simulink model "C172S_HeadingHold_V1"  (R2026a)
settings: Solver=ode4  StartTime=0  StopTime=100  FixedStep=0.01
InitFcn:
  | hh1Data = c172sLateralDirectionalData();
  | [~,hh1Plant] = c172sLateralDirectionalPlant(hh1Data);
  | hh1YawController = c172sYawDamperData();
  | hh1RudderActuator = c172sRudderActuatorData();
  | hh1RollController = c172sRollAttitudeControllerData();
  | hh1AileronActuator = c172sAileronActuatorData();
  | hh1HeadingSensor = c172sHeadingSensorData();
  | hh1HeadingController = c172sHeadingHoldControllerData();
  | if ~strcmp(hh1Data.model.version,hh1HeadingController.requiredPlantVersion), error('HH V1 plant dependency mismatch.'); end
  | if ~strcmp(hh1YawController.artifactRevision,hh1HeadingController.requiredYawDamperRevision), error('HH V1 yaw-controller dependency mismatch.'); end
  | if ~strcmp(hh1RudderActuator.artifactRevision,hh1HeadingController.requiredRudderAuditRevision), error('HH V1 rudder-audit dependency mismatch.'); end
  | if ~strcmp(hh1AileronActuator.artifactRevision,hh1HeadingController.requiredAileronAuditRevision), error('HH V1 aileron-audit dependency mismatch.'); end
  | if ~strcmp(hh1RollController.artifactRevision,hh1HeadingController.requiredRollControllerRevision), error('HH V1 roll-controller dependency mismatch.'); end
  | if ~strcmp(hh1HeadingSensor.artifactRevision,hh1HeadingController.requiredHeadingSensorRevision), error('HH V1 heading-sensor dependency mismatch.'); end
  | A_hh1 = hh1Plant.A; B_hh1 = hh1Plant.B;
  | C_hh1 = hh1Plant.C; D_hh1 = hh1Plant.D;
  | Kphi_hh1 = hh1RollController.bankProportionalGain;
  | Ki_hh1 = hh1RollController.bankIntegralGain_per_s;
  | Kp_hh1 = hh1RollController.rollRateGain_s;
  | Tcmd_hh1 = hh1RollController.commandFilterTimeConstant_s;
  | Kr_hh1 = hh1YawController.rudderGain_s;
  | Tw_hh1 = hh1YawController.washoutTimeConstant_s;
  | TsRudder_hh1 = hh1RudderActuator.sensor.filterTimeConstant_s;
  | tauRudder_hh1 = hh1RudderActuator.dynamics.timeConstant_s;
  | TsRoll_hh1 = hh1AileronActuator.sensor.filterTimeConstant_s;
  | tauAileron_hh1 = hh1AileronActuator.dynamics.timeConstant_s;
  | Tt_hh1 = hh1AileronActuator.antiWindup.trackingTimeConstant_s;
  | delaySampleTime_hh1 = hh1AileronActuator.sensor.nominalDelay_s;
  | Kpsi_hh1 = hh1HeadingController.headingErrorGain;
  | TsHeading_hh1 = hh1HeadingSensor.filterTimeConstant_s;
  | headingDelaySampleTime_hh1 = hh1HeadingSensor.nominalDelay_s/5;
  | bankCommandLower_hh1_rad = -deg2rad(hh1HeadingController.bankCommandAuthority_deg);
  | bankCommandUpper_hh1_rad = deg2rad(hh1HeadingController.bankCommandAuthority_deg);
  | autoAileronLower_hh1_rad = hh1AileronActuator.authority.lowerLimit_rad;
  | autoAileronUpper_hh1_rad = hh1AileronActuator.authority.upperLimit_rad;
  | aileronRateLower_hh1_radps = -deg2rad(hh1AileronActuator.dynamics.rateLimit_degps);
  | aileronRateUpper_hh1_radps = deg2rad(hh1AileronActuator.dynamics.rateLimit_degps);
  | totalAileronLower_hh1_rad = hh1AileronActuator.physicalTravel.lowerLimit_rad;
  | totalAileronUpper_hh1_rad = hh1AileronActuator.physicalTravel.upperLimit_rad;
  | autoRudderLower_hh1_rad = hh1RudderActuator.authority.lowerLimit_rad;
  | autoRudderUpper_hh1_rad = hh1RudderActuator.authority.upperLimit_rad;
  | rudderRateLower_hh1_radps = -deg2rad(hh1RudderActuator.dynamics.rateLimit_degps);
  | rudderRateUpper_hh1_radps = deg2rad(hh1RudderActuator.dynamics.rateLimit_degps);
  | totalRudderLower_hh1_rad = hh1RudderActuator.physicalTravel.lowerLimit_rad;
  | totalRudderUpper_hh1_rad = hh1RudderActuator.physicalTravel.upperLimit_rad;
  | if ~exist('headingCommand_hh1_rad','var'), headingCommand_hh1_rad = deg2rad(30); end
  | if ~exist('headingBias_hh1_rad','var'), headingBias_hh1_rad = 0; end
  | if ~exist('headingNoiseAmplitude_hh1_rad','var'), headingNoiseAmplitude_hh1_rad = 0; end
  | if ~exist('headingNoiseFrequency_hh1_radps','var'), headingNoiseFrequency_hh1_radps = 0.8; end
  | if ~exist('pilotAileronBias_hh1_rad','var'), pilotAileronBias_hh1_rad = 0; end
  | if ~exist('pilotAileronPulse_hh1_rad','var'), pilotAileronPulse_hh1_rad = 0; end
  | if ~exist('pilotRudderBias_hh1_rad','var'), pilotRudderBias_hh1_rad = 0; end
  | if ~exist('pilotRudderPulse_hh1_rad','var'), pilotRudderPulse_hh1_rad = 0; end
  | if ~exist('aileronPulseStart_hh1_s','var'), aileronPulseStart_hh1_s = 5; end
  | if ~exist('aileronPulseEnd_hh1_s','var'), aileronPulseEnd_hh1_s = 6; end
  | if ~exist('rudderPulseStart_hh1_s','var'), rudderPulseStart_hh1_s = 5; end
  | if ~exist('rudderPulseEnd_hh1_s','var'), rudderPulseEnd_hh1_s = 6; end
  | if ~exist('pNoiseAmplitude_hh1_radps','var'), pNoiseAmplitude_hh1_radps = 0; end
  | if ~exist('pNoiseFrequency_hh1_radps','var'), pNoiseFrequency_hh1_radps = 50; end
  | if ~exist('phiNoiseAmplitude_hh1_rad','var'), phiNoiseAmplitude_hh1_rad = 0; end
  | if ~exist('phiNoiseFrequency_hh1_radps','var'), phiNoiseFrequency_hh1_radps = 5; end
  | if ~exist('yawNoiseAmplitude_hh1_radps','var'), yawNoiseAmplitude_hh1_radps = 0; end
  | if ~exist('yawNoiseFrequency_hh1_radps','var'), yawNoiseFrequency_hh1_radps = 50; end
  | if ~exist('antiWindupEnable_hh1','var'), antiWindupEnable_hh1 = 1; end
  | if ~exist('x0_hh1','var'), x0_hh1 = zeros(5,1); end
  | if ~exist('rDelay0_hh1_radps','var'), rDelay0_hh1_radps = x0_hh1(3); end
  | if ~exist('pDelay0_hh1_radps','var'), pDelay0_hh1_radps = x0_hh1(2); end
  | if ~exist('phiDelay0_hh1_rad','var'), phiDelay0_hh1_rad = x0_hh1(4); end
  | if ~exist('rSensor0_hh1_radps','var'), rSensor0_hh1_radps = 0; end
  | if ~exist('xw0_hh1_radps','var'), xw0_hh1_radps = 0; end
  | if ~exist('deltaRAuto0_hh1_rad','var'), deltaRAuto0_hh1_rad = 0; end
  | if ~exist('pSensor0_hh1_radps','var'), pSensor0_hh1_radps = 0; end
  | if ~exist('phiSensor0_hh1_rad','var'), phiSensor0_hh1_rad = 0; end
  | if ~exist('psiDelay0_hh1_rad','var'), psiDelay0_hh1_rad = x0_hh1(5); end
  | if ~exist('psiSensor0_hh1_rad','var'), psiSensor0_hh1_rad = x0_hh1(5)+headingBias_hh1_rad; end
  | if ~exist('xi0_hh1_rad_s','var'), xi0_hh1_rad_s = 0; end
  | if ~exist('deltaAAuto0_hh1_rad','var'), deltaAAuto0_hh1_rad = 0; end
  | if ~exist('filteredCommand0_hh1_rad','var'), filteredCommand0_hh1_rad = 0; end
undefined symbols (not defined in the file or in its folder): aileronPulseEnd_hh1_s, aileronPulseStart_hh1_s, antiWindupEnable_hh1, deltaAAuto0_hh1_rad, deltaRAuto0_hh1_rad, filteredCommand0_hh1_rad, headingBias_hh1_rad, headingNoiseAmplitude_hh1_rad, headingNoiseFrequency_hh1_radps, pDelay0_hh1_radps, phiDelay0_hh1_rad, phiNoiseAmplitude_hh1_rad, phiNoiseFrequency_hh1_radps, phiSensor0_hh1_rad, pilotAileronBias_hh1_rad, pilotAileronPulse_hh1_rad, pilotRudderBias_hh1_rad, pilotRudderPulse_hh1_rad, pNoiseAmplitude_hh1_radps, pNoiseFrequency_hh1_radps, pSensor0_hh1_radps, psiDelay0_hh1_rad, psiSensor0_hh1_rad, rDelay0_hh1_radps, rSensor0_hh1_radps, rudderPulseEnd_hh1_s, rudderPulseStart_hh1_s, x0_hh1, xi0_hh1_rad_s, xw0_hh1_radps, yawNoiseAmplitude_hh1_radps, yawNoiseFrequency_hh1_radps
settings Model: Creator=Shahi  LastModifiedBy=Shahi

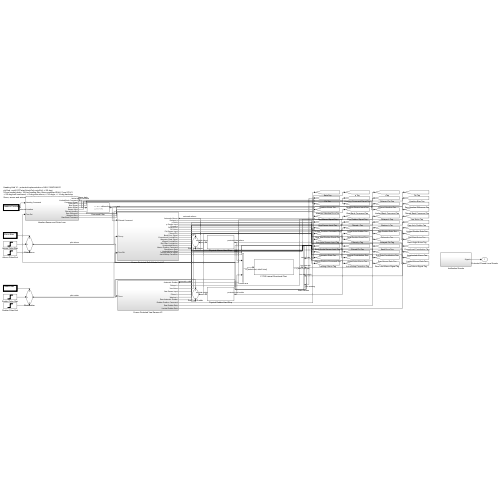
[thumbnail: Simulink's stored preview of the top-level diagram]
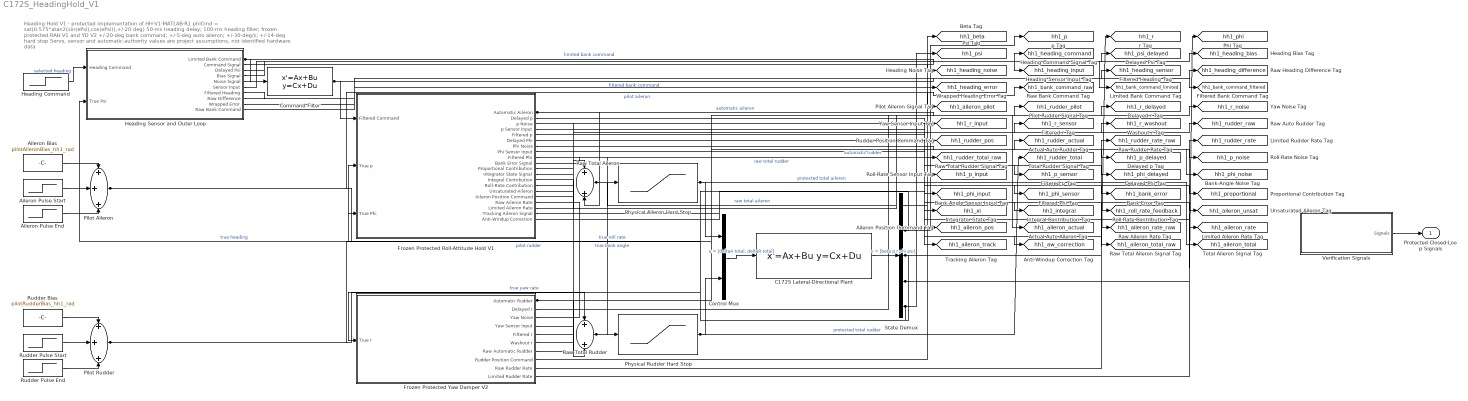
== system C172S_HeadingHold_V1 ==
  note: Heading Hold V1 - protected implementation of HH-V1-MATLAB-R1
      | phiCmd = sat(0.575*atan2(sin(ePsi),cos(ePsi)),+/-20 deg)
      | 50-ms heading delay; 100-ms heading filter; frozen protected RAH V1 and YD V2
      | +/-20-deg bank command; +/-5-deg auto aileron; +/-30-deg/s; +/-14-deg hard stop
      | Servo, sensor and automatic-authority values are project assumptions, not identified hardware data
  Aileron Bias : Constant  Value=pilotAileronBias_hh1_rad
  Aileron Pulse End : Step  Time=aileronPulseEnd_hh1_s  FinalValue=-pilotAileronPulse_hh1_rad  SampleTime=0
  Aileron Pulse Start : Step  Time=aileronPulseStart_hh1_s  FinalValue=pilotAileronPulse_hh1_rad  SampleTime=0
  C172S Lateral-Directional Plant : StateSpace  A=A_hh1  B=B_hh1  C=C_hh1  D=D_hh1  InitialCondition=x0_hh1
  Command Filter : StateSpace  A=-1/Tcmd_hh1  B=1/Tcmd_hh1  D=0  InitialCondition=filteredCommand0_hh1_rad
  Control Mux : Mux  Inputs=2
  Frozen Protected Roll-Attitude Hold V1 : Subsystem
  Frozen Protected Yaw Damper V2 : Subsystem
  Heading Command : Step  Time=0  FinalValue=headingCommand_hh1_rad  SampleTime=0
  Heading Sensor and Outer Loop : Subsystem
  Physical Aileron Hard Stop : Saturate  UpperLimit=totalAileronUpper_hh1_rad  LowerLimit=totalAileronLower_hh1_rad
  Physical Rudder Hard Stop : Saturate  UpperLimit=totalRudderUpper_hh1_rad  LowerLimit=totalRudderLower_hh1_rad
  Pilot Aileron : Sum  Inputs=+++
  Pilot Rudder : Sum  Inputs=+++
  Raw Total Aileron : Sum
  Raw Total Rudder : Sum
  Rudder Bias : Constant  Value=pilotRudderBias_hh1_rad
  Rudder Pulse End : Step  Time=rudderPulseEnd_hh1_s  FinalValue=-pilotRudderPulse_hh1_rad  SampleTime=0
  Rudder Pulse Start : Step  Time=rudderPulseStart_hh1_s  FinalValue=pilotRudderPulse_hh1_rad  SampleTime=0
  State Demux : Demux  Outputs=5
  Verification Signals : Subsystem
  Protected Closed-Loop Signals : Outport
  tag scope: hh1_aileron_actual=global, hh1_aileron_pilot=global, hh1_aileron_pos=global, hh1_aileron_rate=global, hh1_aileron_rate_raw=global, hh1_aileron_total=global, hh1_aileron_total_raw=global, hh1_aileron_track=global, hh1_aileron_unsat=global, hh1_aw_correction=global, hh1_bank_command_filtered=global, hh1_bank_command_limited=global, hh1_bank_command_raw=global, hh1_bank_error=global, hh1_beta=global, hh1_heading_bias=global, hh1_heading_command=global, hh1_heading_difference=global, hh1_heading_error=global, hh1_heading_input=global, hh1_heading_noise=global, hh1_heading_sensor=global, hh1_integral=global, hh1_p=global, hh1_p_delayed=global, hh1_p_input=global, hh1_p_noise=global, hh1_p_sensor=global, hh1_phi=global, hh1_phi_delayed=global, hh1_phi_input=global, hh1_phi_noise=global, hh1_phi_sensor=global, hh1_proportional=global, hh1_psi=global, hh1_psi_delayed=global, hh1_r=global, hh1_r_delayed=global, hh1_r_input=global, hh1_r_noise=global, hh1_r_sensor=global, hh1_r_washout=global, hh1_roll_rate_feedback=global, hh1_rudder_actual=global, hh1_rudder_pilot=global, hh1_rudder_pos=global, hh1_rudder_rate=global, hh1_rudder_rate_raw=global, hh1_rudder_raw=global, hh1_rudder_total=global, hh1_rudder_total_raw=global, hh1_xi=global
  wires:
  Heading Command/1 -> Heading Sensor and Outer Loop/1(Heading Command)  "selected heading"
  Heading Sensor and Outer Loop/1(Limited Bank Command) -> Command Filter/1, [hh1_bank_command_limited]  "limited bank command"
  Command Filter/1 -> Frozen Protected Roll-Attitude Hold V1/1(Filtered Command), [hh1_bank_command_filtered]  "filtered bank command"
  Aileron Bias/1 -> Pilot Aileron/1
  Aileron Pulse Start/1 -> Pilot Aileron/2
  Aileron Pulse End/1 -> Pilot Aileron/3
  Rudder Bias/1 -> Pilot Rudder/1
  Rudder Pulse Start/1 -> Pilot Rudder/2
  Rudder Pulse End/1 -> Pilot Rudder/3
  Pilot Aileron/1 -> Raw Total Aileron/1, [hh1_aileron_pilot]  "pilot aileron"
  Frozen Protected Roll-Attitude Hold V1/1(Automatic Aileron) -> Raw Total Aileron/2, [hh1_aileron_actual]  "automatic aileron"
  Raw Total Aileron/1 -> Physical Aileron Hard Stop/1, [hh1_aileron_total_raw]  "raw total aileron"
  Physical Aileron Hard Stop/1 -> Control Mux/1, [hh1_aileron_total]  "protected total aileron"
  Pilot Rudder/1 -> Raw Total Rudder/1, [hh1_rudder_pilot]  "pilot rudder"
  Frozen Protected Yaw Damper V2/1(Automatic Rudder) -> Raw Total Rudder/2, [hh1_rudder_actual]  "automatic rudder"
  Raw Total Rudder/1 -> Physical Rudder Hard Stop/1, [hh1_rudder_total_raw]  "raw total rudder"
  Physical Rudder Hard Stop/1 -> Control Mux/2, [hh1_rudder_total]  "protected total rudder"
  Control Mux/1 -> C172S Lateral-Directional Plant/1  "u = [deltaA total, deltaR total]"
  C172S Lateral-Directional Plant/1 -> State Demux/1  "x = [beta p r phi psi]"
  State Demux/2 -> Frozen Protected Roll-Attitude Hold V1/2(True p), [hh1_p]  "true roll rate"
  State Demux/4 -> Frozen Protected Roll-Attitude Hold V1/3(True Phi), [hh1_phi]  "true bank angle"
  State Demux/3 -> Frozen Protected Yaw Damper V2/1(True r), [hh1_r]  "true yaw rate"
  State Demux/5 -> Heading Sensor and Outer Loop/2(True Psi), [hh1_psi]  "true heading"
  Verification Signals/1(Signals) -> Protected Closed-Loop Signals/1
  State Demux/1 -> [hh1_beta]
  Heading Sensor and Outer Loop/2(Command Signal) -> [hh1_heading_command]
  Heading Sensor and Outer Loop/3(Delayed Psi) -> [hh1_psi_delayed]
  Heading Sensor and Outer Loop/4(Bias Signal) -> [hh1_heading_bias]
  Heading Sensor and Outer Loop/5(Noise Signal) -> [hh1_heading_noise]
  Heading Sensor and Outer Loop/6(Sensor Input) -> [hh1_heading_input]
  Heading Sensor and Outer Loop/7(Filtered Heading) -> [hh1_heading_sensor]
  Heading Sensor and Outer Loop/8(Raw Difference) -> [hh1_heading_difference]
  Heading Sensor and Outer Loop/9(Wrapped Error) -> [hh1_heading_error]
  Heading Sensor and Outer Loop/10(Raw Bank Command) -> [hh1_bank_command_raw]
  Frozen Protected Yaw Damper V2/2(Delayed r) -> [hh1_r_delayed]
  Frozen Protected Yaw Damper V2/3(Yaw Noise) -> [hh1_r_noise]
  Frozen Protected Yaw Damper V2/4(Yaw Sensor Input) -> [hh1_r_input]
  Frozen Protected Yaw Damper V2/5(Filtered r) -> [hh1_r_sensor]
  Frozen Protected Yaw Damper V2/6(Washout r) -> [hh1_r_washout]
  Frozen Protected Yaw Damper V2/7(Raw Automatic Rudder) -> [hh1_rudder_raw]
  Frozen Protected Yaw Damper V2/8(Rudder Position Command) -> [hh1_rudder_pos]
  Frozen Protected Yaw Damper V2/9(Raw Rudder Rate) -> [hh1_rudder_rate_raw]
  Frozen Protected Yaw Damper V2/10(Limited Rudder Rate) -> [hh1_rudder_rate]
  Frozen Protected Roll-Attitude Hold V1/2(Delayed p) -> [hh1_p_delayed]
  Frozen Protected Roll-Attitude Hold V1/3(p Noise) -> [hh1_p_noise]
  Frozen Protected Roll-Attitude Hold V1/4(p Sensor Input) -> [hh1_p_input]
  Frozen Protected Roll-Attitude Hold V1/5(Filtered p) -> [hh1_p_sensor]
  Frozen Protected Roll-Attitude Hold V1/6(Delayed Phi) -> [hh1_phi_delayed]
  Frozen Protected Roll-Attitude Hold V1/7(Phi Noise) -> [hh1_phi_noise]
  Frozen Protected Roll-Attitude Hold V1/8(Phi Sensor Input) -> [hh1_phi_input]
  Frozen Protected Roll-Attitude Hold V1/9(Filtered Phi) -> [hh1_phi_sensor]
  Frozen Protected Roll-Attitude Hold V1/10(Bank Error Signal) -> [hh1_bank_error]
  Frozen Protected Roll-Attitude Hold V1/11(Proportional Contribution) -> [hh1_proportional]
  Frozen Protected Roll-Attitude Hold V1/12(Integrator State Signal) -> [hh1_xi]
  Frozen Protected Roll-Attitude Hold V1/13(Integral Contribution) -> [hh1_integral]
  Frozen Protected Roll-Attitude Hold V1/14(Roll-Rate Contribution) -> [hh1_roll_rate_feedback]
  Frozen Protected Roll-Attitude Hold V1/15(Unsaturated Aileron) -> [hh1_aileron_unsat]
  Frozen Protected Roll-Attitude Hold V1/16(Aileron Position Command) -> [hh1_aileron_pos]
  Frozen Protected Roll-Attitude Hold V1/17(Raw Aileron Rate) -> [hh1_aileron_rate_raw]
  Frozen Protected Roll-Attitude Hold V1/18(Limited Aileron Rate) -> [hh1_aileron_rate]
  Frozen Protected Roll-Attitude Hold V1/19(Tracking Aileron Signal) -> [hh1_aileron_track]
  Frozen Protected Roll-Attitude Hold V1/20(Anti-Windup Correction) -> [hh1_aw_correction]

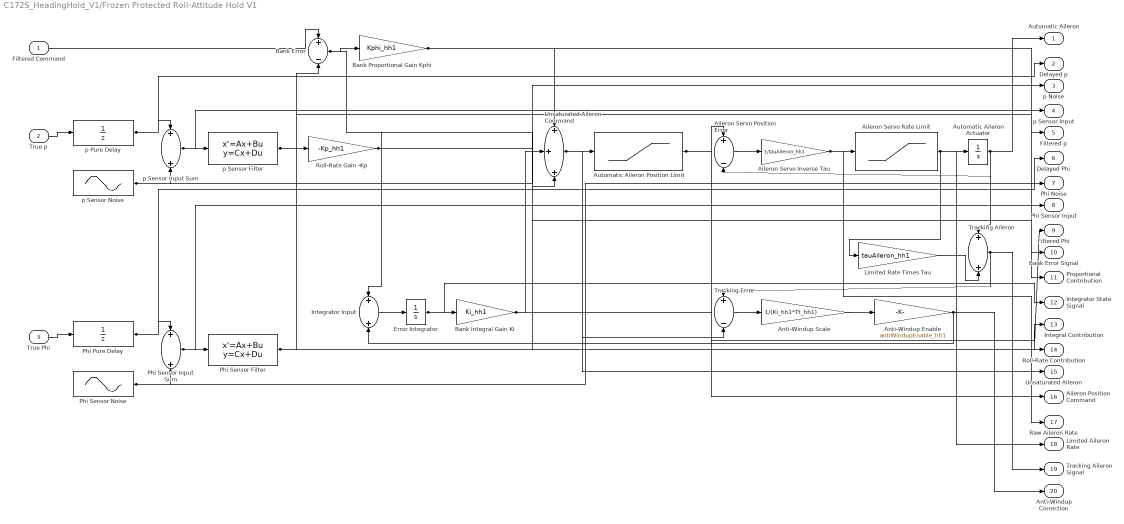
== system C172S_HeadingHold_V1/Frozen Protected Roll-Attitude Hold V1 ==
  Filtered Command : Inport
  True p : Inport  Port=2
  True Phi : Inport  Port=3
  Aileron Servo Inverse Tau : Gain  Gain=1/tauAileron_hh1
  Aileron Servo Position Error : Sum  Inputs=+-
  Aileron Servo Rate Limit : Saturate  UpperLimit=aileronRateUpper_hh1_radps  LowerLimit=aileronRateLower_hh1_radps
  Anti-Windup Enable : Gain  Gain=antiWindupEnable_hh1
  Anti-Windup Scale : Gain  Gain=1/(Ki_hh1*Tt_hh1)
  Automatic Aileron Actuator : Integrator  InitialCondition=deltaAAuto0_hh1_rad
  Automatic Aileron Position Limit : Saturate  UpperLimit=autoAileronUpper_hh1_rad  LowerLimit=autoAileronLower_hh1_rad
  Bank Error : Sum  Inputs=+-
  Bank Integral Gain Ki : Gain  Gain=Ki_hh1
  Bank Proportional Gain Kphi : Gain  Gain=Kphi_hh1
  Error Integrator : Integrator  InitialCondition=xi0_hh1_rad_s
  Integrator Input : Sum
  Limited Rate Times Tau : Gain  Gain=tauAileron_hh1
  Phi Pure Delay : UnitDelay  InitialCondition=phiDelay0_hh1_rad  SampleTime=delaySampleTime_hh1
  Phi Sensor Filter : StateSpace  A=-1/TsRoll_hh1  B=1/TsRoll_hh1  D=0  InitialCondition=phiSensor0_hh1_rad
  Phi Sensor Input Sum : Sum
  Phi Sensor Noise : Sin  Amplitude=phiNoiseAmplitude_hh1_rad  Frequency=phiNoiseFrequency_hh1_radps  SampleTime=0
  Roll-Rate Gain -Kp : Gain  Gain=-Kp_hh1
  Tracking Aileron : Sum
  Tracking Error : Sum  Inputs=+-
  Unsaturated Aileron Command : Sum  Inputs=+++
  p Pure Delay : UnitDelay  InitialCondition=pDelay0_hh1_radps  SampleTime=delaySampleTime_hh1
  p Sensor Filter : StateSpace  A=-1/TsRoll_hh1  B=1/TsRoll_hh1  D=0  InitialCondition=pSensor0_hh1_radps
  p Sensor Input Sum : Sum
  p Sensor Noise : Sin  Amplitude=pNoiseAmplitude_hh1_radps  Frequency=pNoiseFrequency_hh1_radps  SampleTime=0
  Automatic Aileron : Outport
  Delayed p : Outport  Port=2
  p Noise : Outport  Port=3
  p Sensor Input : Outport  Port=4
  Filtered p : Outport  Port=5
  Delayed Phi : Outport  Port=6
  Phi Noise : Outport  Port=7
  Phi Sensor Input : Outport  Port=8
  Filtered Phi : Outport  Port=9
  Bank Error Signal : Outport  Port=10
  Proportional Contribution : Outport  Port=11
  Integrator State Signal : Outport  Port=12
  Integral Contribution : Outport  Port=13
  Roll-Rate Contribution : Outport  Port=14
  Unsaturated Aileron : Outport  Port=15
  Aileron Position Command : Outport  Port=16
  Raw Aileron Rate : Outport  Port=17
  Limited Aileron Rate : Outport  Port=18
  Tracking Aileron Signal : Outport  Port=19
  Anti-Windup Correction : Outport  Port=20
  wires:
  True p/1 -> p Pure Delay/1
  p Pure Delay/1 -> p Sensor Input Sum/1, Delayed p/1
  p Sensor Noise/1 -> p Sensor Input Sum/2, p Noise/1
  p Sensor Input Sum/1 -> p Sensor Filter/1, p Sensor Input/1
  p Sensor Filter/1 -> Roll-Rate Gain -Kp/1, Filtered p/1
  True Phi/1 -> Phi Pure Delay/1
  Phi Pure Delay/1 -> Phi Sensor Input Sum/1, Delayed Phi/1
  Phi Sensor Noise/1 -> Phi Sensor Input Sum/2, Phi Noise/1
  Phi Sensor Input Sum/1 -> Phi Sensor Filter/1, Phi Sensor Input/1
  Filtered Command/1 -> Bank Error/1
  Phi Sensor Filter/1 -> Bank Error/2, Filtered Phi/1
  Bank Error/1 -> Bank Proportional Gain Kphi/1, Integrator Input/1, Bank Error Signal/1
  Integrator Input/1 -> Error Integrator/1
  Error Integrator/1 -> Bank Integral Gain Ki/1, Integrator State Signal/1
  Bank Proportional Gain Kphi/1 -> Unsaturated Aileron Command/1, Proportional Contribution/1
  Bank Integral Gain Ki/1 -> Unsaturated Aileron Command/2, Integral Contribution/1
  Roll-Rate Gain -Kp/1 -> Unsaturated Aileron Command/3, Roll-Rate Contribution/1
  Unsaturated Aileron Command/1 -> Automatic Aileron Position Limit/1, Tracking Error/2, Unsaturated Aileron/1
  Automatic Aileron Position Limit/1 -> Aileron Servo Position Error/1, Aileron Position Command/1
  Automatic Aileron Actuator/1 -> Aileron Servo Position Error/2, Tracking Aileron/1, Automatic Aileron/1
  Aileron Servo Position Error/1 -> Aileron Servo Inverse Tau/1
  Aileron Servo Inverse Tau/1 -> Aileron Servo Rate Limit/1, Raw Aileron Rate/1
  Aileron Servo Rate Limit/1 -> Automatic Aileron Actuator/1, Limited Rate Times Tau/1, Limited Aileron Rate/1
  Limited Rate Times Tau/1 -> Tracking Aileron/2
  Tracking Aileron/1 -> Tracking Error/1, Tracking Aileron Signal/1
  Tracking Error/1 -> Anti-Windup Scale/1
  Anti-Windup Scale/1 -> Anti-Windup Enable/1
  Anti-Windup Enable/1 -> Integrator Input/2, Anti-Windup Correction/1

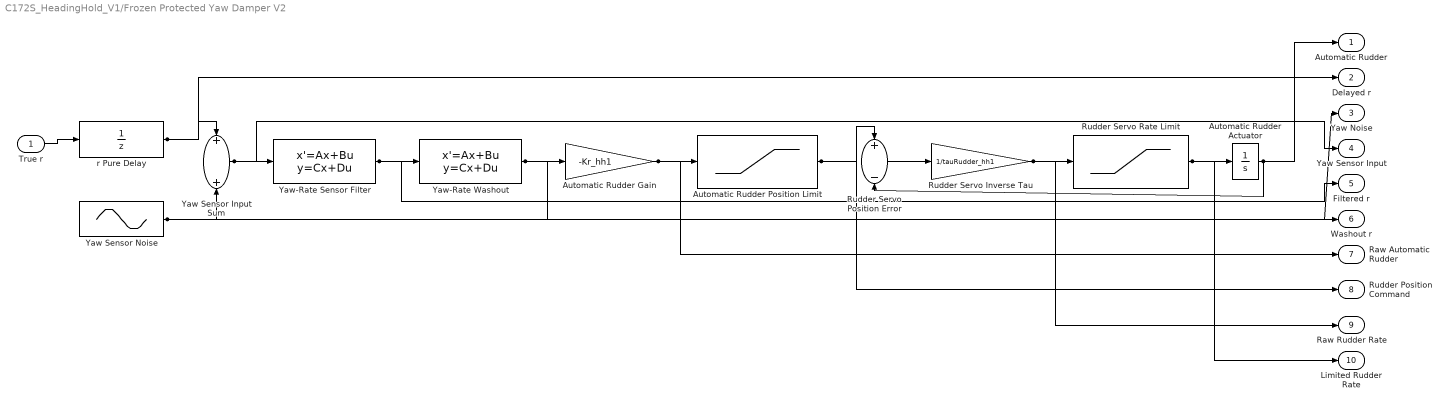
== system C172S_HeadingHold_V1/Frozen Protected Yaw Damper V2 ==
  True r : Inport
  Automatic Rudder Actuator : Integrator  InitialCondition=deltaRAuto0_hh1_rad
  Automatic Rudder Gain : Gain  Gain=-Kr_hh1
  Automatic Rudder Position Limit : Saturate  UpperLimit=autoRudderUpper_hh1_rad  LowerLimit=autoRudderLower_hh1_rad
  Rudder Servo Inverse Tau : Gain  Gain=1/tauRudder_hh1
  Rudder Servo Position Error : Sum  Inputs=+-
  Rudder Servo Rate Limit : Saturate  UpperLimit=rudderRateUpper_hh1_radps  LowerLimit=rudderRateLower_hh1_radps
  Yaw Sensor Input Sum : Sum
  Yaw Sensor Noise : Sin  Amplitude=yawNoiseAmplitude_hh1_radps  Frequency=yawNoiseFrequency_hh1_radps  SampleTime=0
  Yaw-Rate Sensor Filter : StateSpace  A=-1/TsRudder_hh1  B=1/TsRudder_hh1  D=0  InitialCondition=rSensor0_hh1_radps
  Yaw-Rate Washout : StateSpace  A=-1/Tw_hh1  B=1/Tw_hh1  C=-1  InitialCondition=xw0_hh1_radps
  r Pure Delay : UnitDelay  InitialCondition=rDelay0_hh1_radps  SampleTime=delaySampleTime_hh1
  Automatic Rudder : Outport
  Delayed r : Outport  Port=2
  Yaw Noise : Outport  Port=3
  Yaw Sensor Input : Outport  Port=4
  Filtered r : Outport  Port=5
  Washout r : Outport  Port=6
  Raw Automatic Rudder : Outport  Port=7
  Rudder Position Command : Outport  Port=8
  Raw Rudder Rate : Outport  Port=9
  Limited Rudder Rate : Outport  Port=10
  wires:
  True r/1 -> r Pure Delay/1
  r Pure Delay/1 -> Yaw Sensor Input Sum/1, Delayed r/1
  Yaw Sensor Noise/1 -> Yaw Sensor Input Sum/2, Yaw Noise/1
  Yaw Sensor Input Sum/1 -> Yaw-Rate Sensor Filter/1, Yaw Sensor Input/1
  Yaw-Rate Sensor Filter/1 -> Yaw-Rate Washout/1, Filtered r/1
  Yaw-Rate Washout/1 -> Automatic Rudder Gain/1, Washout r/1
  Automatic Rudder Gain/1 -> Automatic Rudder Position Limit/1, Raw Automatic Rudder/1
  Automatic Rudder Position Limit/1 -> Rudder Servo Position Error/1, Rudder Position Command/1
  Automatic Rudder Actuator/1 -> Rudder Servo Position Error/2, Automatic Rudder/1
  Rudder Servo Position Error/1 -> Rudder Servo Inverse Tau/1
  Rudder Servo Inverse Tau/1 -> Rudder Servo Rate Limit/1, Raw Rudder Rate/1
  Rudder Servo Rate Limit/1 -> Automatic Rudder Actuator/1, Limited Rudder Rate/1

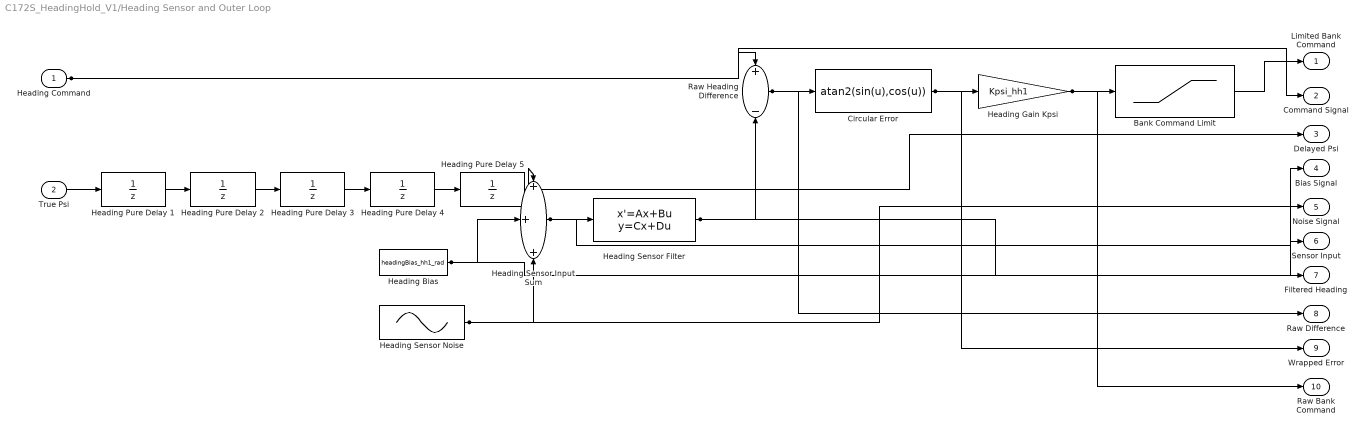
== system C172S_HeadingHold_V1/Heading Sensor and Outer Loop ==
  Heading Command : Inport
  True Psi : Inport  Port=2
  Bank Command Limit : Saturate  UpperLimit=bankCommandUpper_hh1_rad  LowerLimit=bankCommandLower_hh1_rad
  Circular Error : Fcn  Expr=atan2(sin(u),cos(u))
  Heading Bias : Constant  Value=headingBias_hh1_rad
  Heading Gain Kpsi : Gain  Gain=Kpsi_hh1
  Heading Pure Delay {1..5} (5 alike) : UnitDelay  InitialCondition=psiDelay0_hh1_rad  SampleTime=headingDelaySampleTime_hh1
  Heading Sensor Filter : StateSpace  A=-1/TsHeading_hh1  B=1/TsHeading_hh1  D=0  InitialCondition=psiSensor0_hh1_rad
  Heading Sensor Input Sum : Sum  Inputs=+++
  Heading Sensor Noise : Sin  Amplitude=headingNoiseAmplitude_hh1_rad  Frequency=headingNoiseFrequency_hh1_radps  SampleTime=0
  Raw Heading Difference : Sum  Inputs=+-
  Limited Bank Command : Outport
  Command Signal : Outport  Port=2
  Delayed Psi : Outport  Port=3
  Bias Signal : Outport  Port=4
  Noise Signal : Outport  Port=5
  Sensor Input : Outport  Port=6
  Filtered Heading : Outport  Port=7
  Raw Difference : Outport  Port=8
  Wrapped Error : Outport  Port=9
  Raw Bank Command : Outport  Port=10
  wires:
  True Psi/1 -> Heading Pure Delay 1/1
  Heading Pure Delay 1/1 -> Heading Pure Delay 2/1
  Heading Pure Delay 2/1 -> Heading Pure Delay 3/1
  Heading Pure Delay 3/1 -> Heading Pure Delay 4/1
  Heading Pure Delay 4/1 -> Heading Pure Delay 5/1
  Heading Pure Delay 5/1 -> Heading Sensor Input Sum/1, Delayed Psi/1
  Heading Bias/1 -> Heading Sensor Input Sum/2, Bias Signal/1
  Heading Sensor Noise/1 -> Heading Sensor Input Sum/3, Noise Signal/1
  Heading Sensor Input Sum/1 -> Heading Sensor Filter/1, Sensor Input/1
  Heading Command/1 -> Raw Heading Difference/1, Command Signal/1
  Heading Sensor Filter/1 -> Raw Heading Difference/2, Filtered Heading/1
  Raw Heading Difference/1 -> Circular Error/1, Raw Difference/1
  Circular Error/1 -> Heading Gain Kpsi/1, Wrapped Error/1
  Heading Gain Kpsi/1 -> Bank Command Limit/1, Raw Bank Command/1
  Bank Command Limit/1 -> Limited Bank Command/1

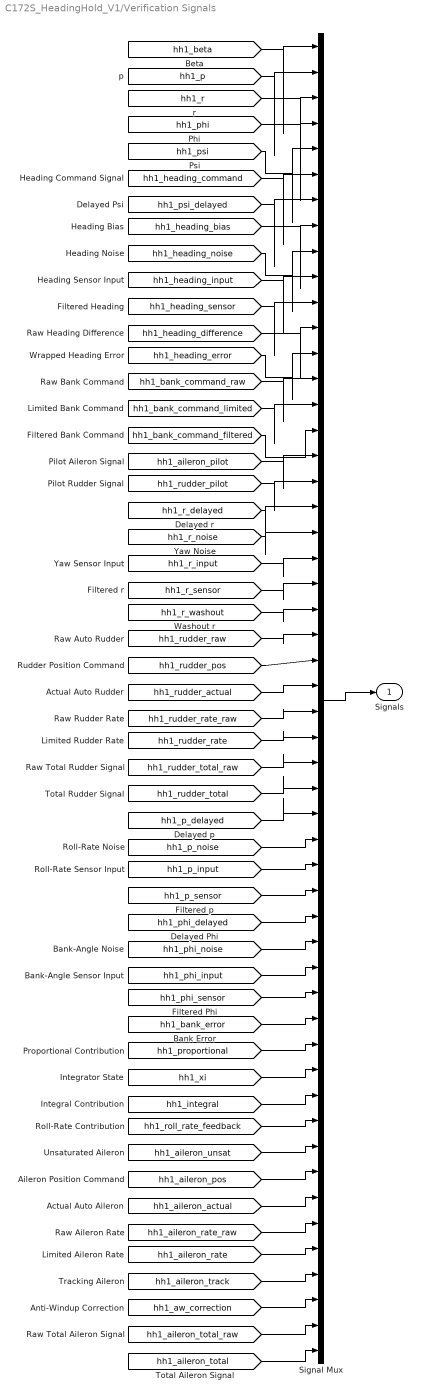
== system C172S_HeadingHold_V1/Verification Signals ==
  Signal Mux : Mux  Inputs=52
  Signals : Outport
  wires:
  [hh1_beta] -> Signal Mux/1
  [hh1_p] -> Signal Mux/2
  [hh1_r] -> Signal Mux/3
  [hh1_phi] -> Signal Mux/4
  [hh1_psi] -> Signal Mux/5
  [hh1_heading_command] -> Signal Mux/6
  [hh1_psi_delayed] -> Signal Mux/7
  [hh1_heading_bias] -> Signal Mux/8
  [hh1_heading_noise] -> Signal Mux/9
  [hh1_heading_input] -> Signal Mux/10
  [hh1_heading_sensor] -> Signal Mux/11
  [hh1_heading_difference] -> Signal Mux/12
  [hh1_heading_error] -> Signal Mux/13
  [hh1_bank_command_raw] -> Signal Mux/14
  [hh1_bank_command_limited] -> Signal Mux/15
  [hh1_bank_command_filtered] -> Signal Mux/16
  [hh1_aileron_pilot] -> Signal Mux/17
  [hh1_rudder_pilot] -> Signal Mux/18
  [hh1_r_delayed] -> Signal Mux/19
  [hh1_r_noise] -> Signal Mux/20
  [hh1_r_input] -> Signal Mux/21
  [hh1_r_sensor] -> Signal Mux/22
  [hh1_r_washout] -> Signal Mux/23
  [hh1_rudder_raw] -> Signal Mux/24
  [hh1_rudder_pos] -> Signal Mux/25
  [hh1_rudder_actual] -> Signal Mux/26
  [hh1_rudder_rate_raw] -> Signal Mux/27
  [hh1_rudder_rate] -> Signal Mux/28
  [hh1_rudder_total_raw] -> Signal Mux/29
  [hh1_rudder_total] -> Signal Mux/30
  [hh1_p_delayed] -> Signal Mux/31
  [hh1_p_noise] -> Signal Mux/32
  [hh1_p_input] -> Signal Mux/33
  [hh1_p_sensor] -> Signal Mux/34
  [hh1_phi_delayed] -> Signal Mux/35
  [hh1_phi_noise] -> Signal Mux/36
  [hh1_phi_input] -> Signal Mux/37
  [hh1_phi_sensor] -> Signal Mux/38
  [hh1_bank_error] -> Signal Mux/39
  [hh1_proportional] -> Signal Mux/40
  [hh1_xi] -> Signal Mux/41
  [hh1_integral] -> Signal Mux/42
  [hh1_roll_rate_feedback] -> Signal Mux/43
  [hh1_aileron_unsat] -> Signal Mux/44
  [hh1_aileron_pos] -> Signal Mux/45
  [hh1_aileron_actual] -> Signal Mux/46
  [hh1_aileron_rate_raw] -> Signal Mux/47
  [hh1_aileron_rate] -> Signal Mux/48
  [hh1_aileron_track] -> Signal Mux/49
  [hh1_aw_correction] -> Signal Mux/50
  [hh1_aileron_total_raw] -> Signal Mux/51
  [hh1_aileron_total] -> Signal Mux/52
  Signal Mux/1 -> Signals/1
